simulink model "Roadsense_SensorFusion"  (R2025b)
settings: Solver=FixedStepDiscrete  StartTime=0.0  StopTime=1.0  FixedStep=RsTsBase  RelTol=1e-3
undefined symbols (not defined in the file or in its folder): RsMaxDetections, RsMaxTracks, RsTsFusion
settings Model: DataDictionary=Roadsense_Data.sldd  Creator=ragur  LastModifiedBy=ragur

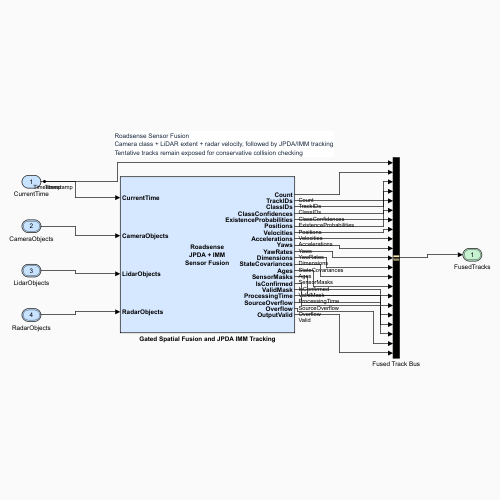
[thumbnail: Simulink's stored preview of the top-level diagram]
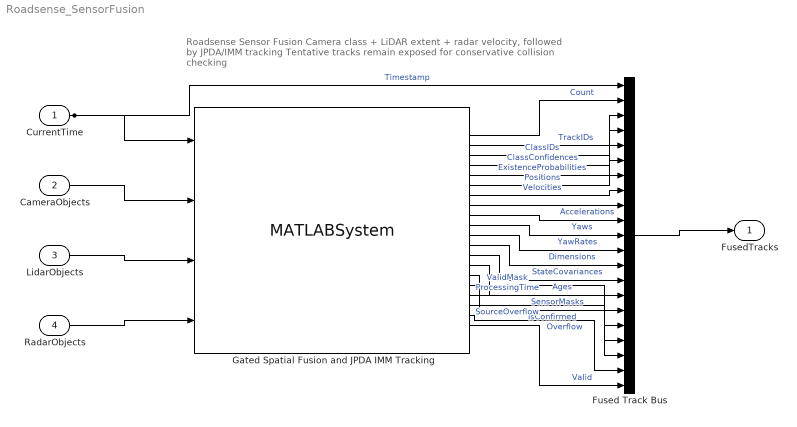
== system Roadsense_SensorFusion ==
  note: Roadsense Sensor Fusion
      | Camera class + LiDAR extent + radar velocity, followed by JPDA/IMM tracking
      | Tentative tracks remain exposed for conservative collision checking
  CurrentTime : Inport  OutDataTypeStr=double  SampleTime=RsTsFusion
  CameraObjects : Inport  Port=2  OutDataTypeStr=Bus: RsCameraObjectListBus  PortDimensions=1  SampleTime=RsTsFusion
  LidarObjects : Inport  Port=3  OutDataTypeStr=Bus: RsLidarObjectListBus  PortDimensions=1  SampleTime=RsTsFusion
  RadarObjects : Inport  Port=4  OutDataTypeStr=Bus: RsRadarObjectListBus  PortDimensions=1  SampleTime=RsTsFusion
  Fused Track Bus : BusCreator  Inputs=21  OutDataTypeStr=Bus: RsFusedTrackListBus
  Gated Spatial Fusion and JPDA IMM Tracking : MATLABSystem  System=RoadsenseSensorFusionSystem  MaxDetections=double(RsMaxDetections)  MaxTracks=double(RsMaxTracks)  NumberClasses=10  CameraLidarGate=RsFusionCameraLidarGate  RadarLidarGate=RsFusionRadarLidarGate  CameraRadarGate=RsFusionCameraRadarGate  AssignmentThreshold=RsFusionTrackAssociationThreshold  ConfirmationProbability=RsFusionConfirmationProbability  DeletionProbability=RsFusionDeletionProbability  DetectionProbability=RsFusionDetectionProbability  SimulateUsing=Interpreted execution
      mask Type: RoadsenseSensorFusionSystem
  FusedTracks : Outport  OutDataTypeStr=Bus: RsFusedTrackListBus
  wires:
  CurrentTime/1 -> Gated Spatial Fusion and JPDA IMM Tracking/1, Fused Track Bus/1  "Timestamp"
  CameraObjects/1 -> Gated Spatial Fusion and JPDA IMM Tracking/2
  LidarObjects/1 -> Gated Spatial Fusion and JPDA IMM Tracking/3
  RadarObjects/1 -> Gated Spatial Fusion and JPDA IMM Tracking/4
  Gated Spatial Fusion and JPDA IMM Tracking/1 -> Fused Track Bus/2  "Count"
  Gated Spatial Fusion and JPDA IMM Tracking/2 -> Fused Track Bus/3  "TrackIDs"
  Gated Spatial Fusion and JPDA IMM Tracking/3 -> Fused Track Bus/4  "ClassIDs"
  Gated Spatial Fusion and JPDA IMM Tracking/4 -> Fused Track Bus/5  "ClassConfidences"
  Gated Spatial Fusion and JPDA IMM Tracking/5 -> Fused Track Bus/6  "ExistenceProbabilities"
  Gated Spatial Fusion and JPDA IMM Tracking/6 -> Fused Track Bus/7  "Positions"
  Gated Spatial Fusion and JPDA IMM Tracking/7 -> Fused Track Bus/8  "Velocities"
  Gated Spatial Fusion and JPDA IMM Tracking/8 -> Fused Track Bus/9  "Accelerations"
  Gated Spatial Fusion and JPDA IMM Tracking/9 -> Fused Track Bus/10  "Yaws"
  Gated Spatial Fusion and JPDA IMM Tracking/10 -> Fused Track Bus/11  "YawRates"
  Gated Spatial Fusion and JPDA IMM Tracking/11 -> Fused Track Bus/12  "Dimensions"
  Gated Spatial Fusion and JPDA IMM Tracking/12 -> Fused Track Bus/13  "StateCovariances"
  Gated Spatial Fusion and JPDA IMM Tracking/13 -> Fused Track Bus/14  "Ages"
  Gated Spatial Fusion and JPDA IMM Tracking/14 -> Fused Track Bus/15  "SensorMasks"
  Gated Spatial Fusion and JPDA IMM Tracking/15 -> Fused Track Bus/16  "IsConfirmed"
  Gated Spatial Fusion and JPDA IMM Tracking/16 -> Fused Track Bus/17  "ValidMask"
  Gated Spatial Fusion and JPDA IMM Tracking/17 -> Fused Track Bus/18  "ProcessingTime"
  Gated Spatial Fusion and JPDA IMM Tracking/18 -> Fused Track Bus/19  "SourceOverflow"
  Gated Spatial Fusion and JPDA IMM Tracking/19 -> Fused Track Bus/20  "Overflow"
  Gated Spatial Fusion and JPDA IMM Tracking/20 -> Fused Track Bus/21  "Valid"
  Fused Track Bus/1 -> FusedTracks/1
